simulink model "ups_control"  (Simulink 10.3)
settings: Solver=ode5  StartTime=0.0  StopTime=t_end  FixedStep=Ts  RelTol=1e-3  EnableMultiTasking=on
values from neighbouring files (symbols this model uses):
  A_r = sysd.a    [ups_controller_design.m]
  B_r = sysd.b    [ups_controller_design.m]
  C_r = sysd.c    [ups_controller_design.m]
  CLinear = 0    [ups_settings.m]
  CNLinear = 1    [ups_settings.m]
  D_r = sysd.d    [ups_controller_design.m]
  f = 60    [run_ups.m]
  K = W/Q    [ups_controller_design.m]
  K_pwm = V_cc/(2*V_sat)    (= 1)    [ups_settings.m]
  T = 1/fa    (= 9.98003992016e-05)    [run_ups.m]
  t_end = 2    [run_ups.m]
  Ts = 1/(100*fa)    (= 9.98003992016e-07)    [run_ups.m]
  u0 = V_cc/2    (= 260)    [ups_settings.m]
  V_cc = 520    [ups_settings.m]
  V_ma = Vo_rms*1.1    (= 139.7)    [ups_settings.m]
  V_mi = Vo_rms*0.9    (= 114.3)    [ups_settings.m]
  Vo_pk = 127*sqrt(2)    [ups_settings.m]
libraries: powerlib_extras x2
settings Model: Creator=Projeto UPS  LastModifiedBy=gkeie
settings DataIOCC: SignalLoggingName=sigsOut
settings DebuggingCC: SaveWithParameterizedLinksMsg=none  SignalResolutionControl=TryResolveAllWithWarning  MultiTaskDSMMsg=warning  MultiTaskCondExecSysMsg=none
settings HardwareCC: TargetUnknown=on

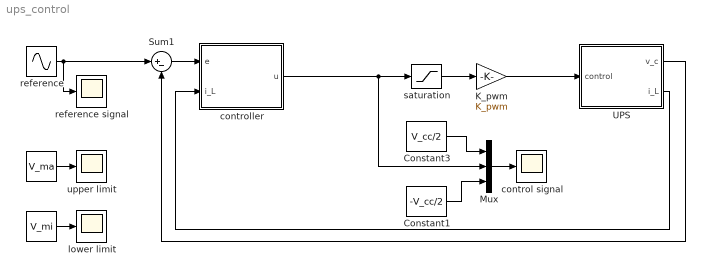
== system ups_control ==
  "            " : Constant  Value=V_ma  SampleTime=-1
  "                                   " : Constant  Value=V_mi  SampleTime=-1
  " K_pwm" : Gain  Gain=K_pwm  SaturateOnIntegerOverflow=on  OutDataTypeStr=Inherit: Same as input  ParamDataTypeStr=Inherit: Same as input
  Constant1 : Constant  Value=-V_cc/2  SampleTime=-1
  Constant3 : Constant  Value=V_cc/2  SampleTime=-1
  Mux : Mux  Inputs=3
  Sum1 : Sum  Inputs=|+-  SaturateOnIntegerOverflow=on
  UPS : Subsystem
  control signal : Scope
  controller : Subsystem
  lower limit : Scope
  reference : Sin  Amplitude=Vo_pk  Frequency=2*pi*f  SampleTime=Ts
  reference signal : Scope
  saturation : Saturate  UpperLimit=u0  LowerLimit=-u0  LinearizeAsGain=off
  upper limit : Scope
  wires:
  reference/1 -> Sum1/1, reference signal/1
  Sum1/1 -> controller/1(e)
  UPS/2(i_L) -> controller/2(i_L)
  UPS/1(v_c) -> Sum1/2
  saturation/1 -> " K_pwm"/1
  " K_pwm"/1 -> UPS/1(control)
  Constant1/1 -> Mux/3
  "            "/1 -> upper limit/1
  Constant3/1 -> Mux/1
  controller/1(u) -> Mux/2, saturation/1
  Mux/1 -> control signal/1
  "                                   "/1 -> lower limit/1

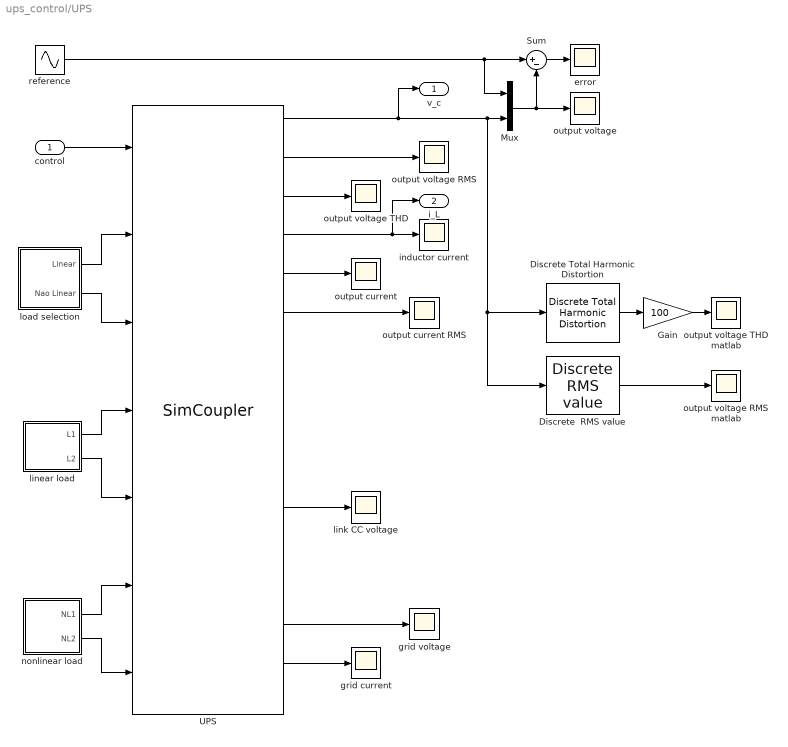
== system ups_control/UPS ==
  control : Inport
  Discrete Total Harmonic Distortion : powerlib_extras/Discrete Measurements/Discrete Total Harmonic Distortion  Freq=f  Ts=Ts
      settings: SourceProductBaseCode=PS
  Discrete  RMS value : powerlib_extras/Discrete Measurements/Discrete  RMS value  Freq=f  Mag_Init=0  Ts=Ts
      settings: SourceProductBaseCode=PS
  Gain : Gain  Gain=100
  Mux : Mux  Inputs=2
  Sum : Sum  Inputs=|+-
  UPS : S-Function  FunctionName=SimCoupler  Parameters='C:\Users\gkeie\Dropbox\backup\ups_guilherme\ups\ups.psimsch'  SFunctionDeploymentMode=off  EnableBusSupport=off
      mask init:
      | c=[0:10:360]*pi/180;
      | x1=cos(c)*30; y1=sin(c)*30+20;
      | x2=cos(c)*30;y2=sin(c)*30-20;
      settings: OpenFcn=PSimDialog('PSimFileEdt','Value','Parameters');  CloseFcn=close(gcf);
      mask Display: plot(-60,-60,60,60,x1,y1,x2,y2)
  error : Scope
  grid current : Scope
  grid voltage : Scope
  inductor current : Scope
  linear load : Subsystem
  link CC voltage : Scope
  load selection : Subsystem
  nonlinear load : Subsystem
  output current : Scope
  output current RMS : Scope
  output voltage : Scope
  output voltage RMS : Scope
  output voltage RMS matlab : Scope
  output voltage THD : Scope
  "output voltage THD matlab    " : Scope
  reference : Sin  Amplitude=Vo_pk  Frequency=2*pi*f  SampleTime=Ts
  v_c : Outport
  i_L : Outport  Port=2
  wires:
  control/1 -> UPS/1
  UPS/1 -> v_c/1, Mux/2, Discrete Total Harmonic Distortion/1, Discrete  RMS value/1
  UPS/6 -> output current RMS/1
  reference/1 -> Mux/1, Sum/1
  UPS/2 -> output voltage RMS/1
  UPS/3 -> output voltage THD/1
  UPS/4 -> i_L/1, inductor current/1
  UPS/5 -> output current/1
  UPS/11 -> link CC voltage/1
  UPS/14 -> grid voltage/1
  UPS/15 -> grid current/1
  Discrete Total Harmonic Distortion/1 -> Gain/1
  Gain/1 -> "output voltage THD matlab    "/1
  Discrete  RMS value/1 -> output voltage RMS matlab/1
  load selection/1(Linear) -> UPS/2
  load selection/2(Nao Linear) -> UPS/3
  linear load/1(L1) -> UPS/4
  linear load/2(L2) -> UPS/5
  nonlinear load/1(NL1) -> UPS/6
  nonlinear load/2(NL2) -> UPS/7
  Sum/1 -> error/1
  Mux/1 -> output voltage/1, Sum/2

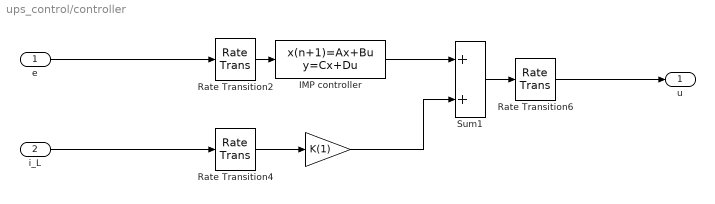
== system ups_control/controller ==
  e : Inport
  i_L : Inport  Port=2
  "         " : Gain  Gain=K(1)  SaturateOnIntegerOverflow=on  OutDataTypeStr=Inherit: Same as input  ParamDataTypeStr=Inherit: Same as input
  IMP controller : DiscreteStateSpace  A=A_r  B=B_r  C=C_r  D=D_r  SampleTime=T
  Rate Transition2 : RateTransition
  Rate Transition4 : RateTransition
  Rate Transition6 : RateTransition
  Sum1 : Sum
  u : Outport
  wires:
  IMP controller/1 -> Sum1/1
  "         "/1 -> Sum1/2
  e/1 -> Rate Transition2/1
  i_L/1 -> Rate Transition4/1
  Rate Transition2/1 -> IMP controller/1
  Rate Transition4/1 -> "         "/1
  Sum1/1 -> Rate Transition6/1
  Rate Transition6/1 -> u/1

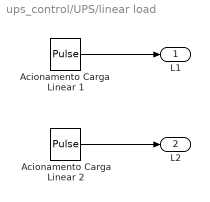
== system ups_control/UPS/linear load ==
  "Acionamento Carga  Linear 1 " : DiscretePulseGenerator  PulseType=Time based  Amplitude=t_end  Period=t_end  PulseWidth=80  PhaseDelay=0.2
  "Acionamento Carga Linear 2 " : DiscretePulseGenerator  PulseType=Time based  Amplitude=t_end  Period=t_end  PulseWidth=40  PhaseDelay=0.6
  L1 : Outport
  L2 : Outport  Port=2
  wires:
  "Acionamento Carga  Linear 1 "/1 -> L1/1
  "Acionamento Carga Linear 2 "/1 -> L2/1

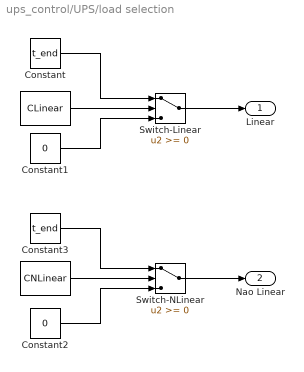
== system ups_control/UPS/load selection ==
  " " : Constant  Value=CLinear  VectorParams1D=off  OutDataTypeStr=boolean  SampleTime=-1
  "  " : Constant  Value=CNLinear  VectorParams1D=off  OutDataTypeStr=boolean  SampleTime=-1
  Constant : Constant  Value=t_end  SampleTime=-1
  Constant1 : Constant  Value=0  SampleTime=-1
  Constant2 : Constant  Value=0  SampleTime=-1
  Constant3 : Constant  Value=t_end  SampleTime=-1
  Switch-Linear : Switch
  Switch-NLinear : Switch
  Linear : Outport
  Nao Linear : Outport  Port=2
  wires:
  Switch-Linear/1 -> Linear/1
  " "/1 -> Switch-Linear/2
  Switch-NLinear/1 -> Nao Linear/1
  "  "/1 -> Switch-NLinear/2
  Constant/1 -> Switch-Linear/1
  Constant2/1 -> Switch-NLinear/3
  Constant3/1 -> Switch-NLinear/1
  Constant1/1 -> Switch-Linear/3

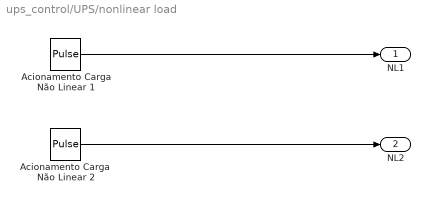
== system ups_control/UPS/nonlinear load ==
  Acionamento Carga  Não Linear 2 : DiscretePulseGenerator  PulseType=Time based  Amplitude=t_end  Period=t_end  PulseWidth=40  PhaseDelay=0.6
  "Acionamento Carga Não Linear 1 " : DiscretePulseGenerator  PulseType=Time based  Amplitude=t_end  Period=t_end  PulseWidth=80  PhaseDelay=0.2
  NL1 : Outport
  NL2 : Outport  Port=2
  wires:
  "Acionamento Carga Não Linear 1 "/1 -> NL1/1
  Acionamento Carga  Não Linear 2/1 -> NL2/1
